simulink model "Reference"  (R2018b)
settings: Solver=ode45  StartTime=0.0  StopTime=2  FixedStep=1e-6  RelTol=1e-9
undefined symbols (not defined in the file or in its folder): alpha_rel, kp1, kp2, kv1, kv2, rad_deg
settings Model: Creator=a.brugnoli  LastModifiedBy=a.brugnoli

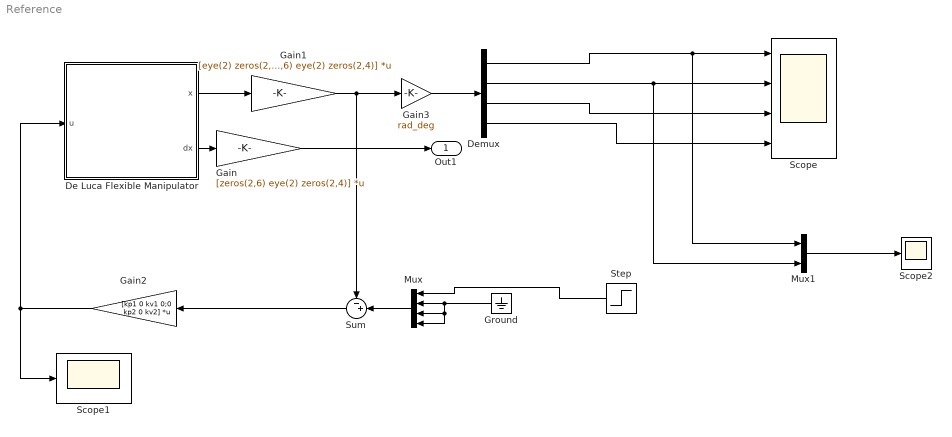
== system Reference ==
  De Luca Flexible Manipulator : Subsystem
  Demux : Demux
  Gain : Gain  Gain=[zeros(2,6) eye(2) zeros(2,4)]  Multiplication=Matrix(K*u) (u vector)
  Gain1 : Gain  Gain=[eye(2) zeros(2,10); zeros(2,6) eye(2) zeros(2,4)]  Multiplication=Matrix(K*u) (u vector)
  Gain2 : Gain  Gain="[kp1 0 kv1 0;0  kp2 0  kv2]"  Multiplication=Matrix(K*u) (u vector)
  Gain3 : Gain  Gain=rad_deg
  Ground : Ground
  Mux : Mux
  Mux1 : Mux  Inputs=2
  Scope : Scope  NumInputPorts=4
  Scope1 : Scope
  Scope2 : Scope
  Step : Step  After=alpha_rel  SampleTime=0
  Sum : Sum  Inputs=-+|
  Out1 : Outport
  wires:
  Demux/4 -> Scope/4
  De Luca Flexible Manipulator/2(dx) -> Gain/1
  Gain1/1 -> Gain3/1, Sum/1
  Demux/1 -> Mux1/1, Scope/1
  Demux/2 -> Mux1/2, Scope/2
  De Luca Flexible Manipulator/1(x) -> Gain1/1
  Gain/1 -> Out1/1
  Demux/3 -> Scope/3
  Step/1 -> Mux/1
  Ground/1 -> Mux/4, Mux/3, Mux/2
  Mux/1 -> Sum/2
  Sum/1 -> Gain2/1
  Gain3/1 -> Demux/1
  Gain2/1 -> De Luca Flexible Manipulator/1(u), Scope1/1
  Mux1/1 -> Scope2/1

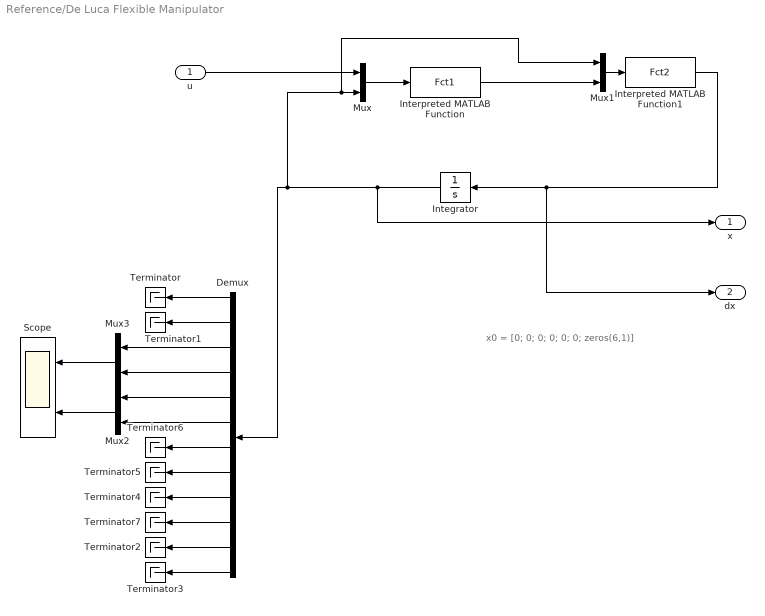
== system Reference/De Luca Flexible Manipulator ==
  note: x0 = [0; 0; 0; 0; 0; 0; zeros(6,1)]
  u : Inport  PortDimensions=2
  Demux : Demux  Outputs=12
  Integrator : Integrator  InitialCondition="[0; pi/2; 0.1; 0.002; 0; 0;  zeros(6,1);]"
  Interpreted MATLAB Function : MATLABFcn  MATLABFcn=Fct1  OutputDimensions=12
  Interpreted MATLAB Function1 : MATLABFcn  MATLABFcn=Fct2  OutputDimensions=12
  Mux : Mux  Inputs=[2 12]
  Mux1 : Mux  Inputs=[12 12]
  Mux2 : Mux  Inputs=2
  Mux3 : Mux  Inputs=2
  Scope : Scope  NumInputPorts=2
  Terminator{,1..7} (8 alike) : Terminator
  x : Outport  PortDimensions=12
  dx : Outport  Port=2  PortDimensions=12
  wires:
  u/1 -> Mux/1
  Interpreted MATLAB Function1/1 -> dx/1, Integrator/1
  Mux/1 -> Interpreted MATLAB Function/1
  Interpreted MATLAB Function/1 -> Mux1/2
  Integrator/1 -> x/1, Demux/1, Mux1/1, Mux/2
  Mux1/1 -> Interpreted MATLAB Function1/1
  Demux/3 -> Mux3/1
  Demux/4 -> Mux3/2
  Demux/5 -> Mux2/1
  Demux/6 -> Mux2/2
  Mux3/1 -> Scope/1
  Mux2/1 -> Scope/2
  Demux/1 -> Terminator/1
  Demux/2 -> Terminator1/1
  Demux/7 -> Terminator6/1
  Demux/8 -> Terminator5/1
  Demux/9 -> Terminator4/1
  Demux/10 -> Terminator7/1
  Demux/11 -> Terminator2/1
  Demux/12 -> Terminator3/1
